simulink model "SecRwLtStCalib"  (R2024b)
settings: Solver=FixedStepDiscrete  StartTime=0.0  StopTime=10.0  FixedStep=0.01  RelTol=1e-3
model workspace (MAT data in the model file):
  KeSMSwAcsMd6SecRwLtStBkReclnUpwdDnwdPos1Max_Val : Simulink.Parameter (value not decoded)
  KeSMSwAcsMd6SecRwLtStBkReclnUpwdDnwdPos1Min_Val : Simulink.Parameter (value not decoded)
  KeSMSwAcsMd6SecRwLtStBkReclnUpwdDnwdPos1_Val : Simulink.Parameter (value not decoded)
  KeSMSwAcsMd6SecRwLtStBkReclnUpwdDnwdPosMax_Val : Simulink.Parameter (value not decoded)
  KeSMSwAcsMd6SecRwLtStBkReclnUpwdDnwdPosMin_Val : Simulink.Parameter (value not decoded)
  KeSMSwAcsMd6SecRwLtStBkReclnUpwdDnwdPos_Val : Simulink.Parameter (value not decoded)
symbols that are objects in the model workspace (value not decoded): KeSMSwAcsMd6SecRwLtStBkReclnUpwdDnwdPos1_Val, KeSMSwAcsMd6SecRwLtStBkReclnUpwdDnwdPos1Max_Val, KeSMSwAcsMd6SecRwLtStBkReclnUpwdDnwdPos1Min_Val, KeSMSwAcsMd6SecRwLtStBkReclnUpwdDnwdPos_Val, KeSMSwAcsMd6SecRwLtStBkReclnUpwdDnwdPosMax_Val, KeSMSwAcsMd6SecRwLtStBkReclnUpwdDnwdPosMin_Val
undefined symbols (not defined in the file or in its folder): KeSMSw4SAcsMd21SecRwLtStBkReclnUpwdDnwdPos_Val, KeSMSw4SAcsMd21SecRwLtStBkReclnUpwdDnwdPosMax_Val, KeSMSw4SAcsMd21SecRwLtStBkReclnUpwdDnwdPosMin_Val, KeSMSw4SAcsMd21SecRwLtStFrwdBkwdPos_Val, KeSMSw4SAcsMd21SecRwLtStFrwdBkwdPosMax_Val, KeSMSw4SAcsMd21SecRwLtStFrwdBkwdPosMin_Val, KeSMSw4SAcsMd21SecRwLtStHdrstFrwdBkwdPos_Val, KeSMSw4SAcsMd21SecRwLtStHdrstFrwdBkwdPosMax_Val, KeSMSw4SAcsMd21SecRwLtStHdrstFrwdBkwdPosMin_Val, KeSMSw4SAcsMd21SecRwLtStHdrstUpwdDnwdPos_Val, KeSMSw4SAcsMd21SecRwLtStHdrstUpwdDnwdPosMax_Val, KeSMSw4SAcsMd21SecRwLtStHdrstUpwdDnwdPosMin_Val, KeSMSw4SAcsMd22SecRwLtStBkReclnUpwdDnwdPos1_Val, KeSMSw4SAcsMd22SecRwLtStBkReclnUpwdDnwdPos2_Val, KeSMSw4SAcsMd22SecRwLtStBkReclnUpwdDnwdPos2Max_Val, KeSMSw4SAcsMd22SecRwLtStBkReclnUpwdDnwdPos2Min_Val, KeSMSw4SAcsMd22SecRwLtStBkReclnUpwdDnwdPosMax_Val, KeSMSw4SAcsMd22SecRwLtStBkReclnUpwdDnwdPosMin_Val, KeSMSw4SAcsMd22SecRwLtStFrwdBkwdPos_Val, KeSMSw4SAcsMd22SecRwLtStFrwdBkwdPosMax_Val, KeSMSw4SAcsMd22SecRwLtStFrwdBkwdPosMin_Val, KeSMSw4SAcsMd22SecRwLtStFtrstUpwdDnwdPos_Val, KeSMSw4SAcsMd22SecRwLtStFtrstUpwdDnwdPosMax_Val, KeSMSw4SAcsMd22SecRwLtStFtrstUpwdDnwdPosMin_Val, KeSMSw4SAcsMd22SecRwLtStHdrstFrwdBkwdPos_Val, KeSMSw4SAcsMd22SecRwLtStHdrstFrwdBkwdPosMax_Val, KeSMSw4SAcsMd22SecRwLtStHdrstFrwdBkwdPosMin_Val, KeSMSw4SAcsMd22SecRwLtStHdrstUpwdDnwdPos_Val, KeSMSw4SAcsMd22SecRwLtStHdrstUpwdDnwdPosMax_Val, KeSMSw4SAcsMd22SecRwLtStHdrstUpwdDnwdPosMin_Val, KeSMSw4SAcsMd22SecRwLtStLegrstOtwdInwdPos_Val, KeSMSw4SAcsMd22SecRwLtStLegrstOtwdInwdPosMax_Val, KeSMSw4SAcsMd22SecRwLtStLegrstOtwdInwdPosMin_Val, KeSMSw4SAcsMd22SecRwLtStLegrstUpwdDnwdPos_Val, KeSMSw4SAcsMd22SecRwLtStLegrstUpwdDnwdPosMax_Val, KeSMSw4SAcsMd22SecRwLtStLegrstUpwdDnwdPosMin_Val, KeSMSw4SAcsMd25SecRwLtStBkReclnUpwdDnwdPos_Val, KeSMSw4SAcsMd25SecRwLtStBkReclnUpwdDnwdPosMax_Val, KeSMSw4SAcsMd25SecRwLtStBkReclnUpwdDnwdPosMin_Val, KeSMSw4SAcsMd25SecRwLtStFrwdBkwdPos_Val, KeSMSw4SAcsMd25SecRwLtStFrwdBkwdPosMax_Val, KeSMSw4SAcsMd25SecRwLtStFrwdBkwdPosMin_Val, KeSMSw4SAcsMd25SecRwLtStHdrstFrwdBkwdPos_Val, KeSMSw4SAcsMd25SecRwLtStHdrstFrwdBkwdPosMax_Val, KeSMSw4SAcsMd25SecRwLtStHdrstFrwdBkwdPosMin_Val, KeSMSw4SAcsMd25SecRwLtStHdrstUpwdDnwdPos_Val, KeSMSw4SAcsMd25SecRwLtStHdrstUpwdDnwdPosMax_Val, KeSMSw4SAcsMd25SecRwLtStHdrstUpwdDnwdPosMin_Val, KeSMSw4SAcsMd26SecRwLtStBkReclnUpwdDnwdPos_Val, KeSMSw4SAcsMd26SecRwLtStBkReclnUpwdDnwdPosMax_Val, KeSMSw4SAcsMd26SecRwLtStBkReclnUpwdDnwdPosMin_Val, KeSMSw4SAcsMd26SecRwLtStFrwdBkwdPos_Val, KeSMSw4SAcsMd26SecRwLtStFrwdBkwdPosMax_Val, KeSMSw4SAcsMd26SecRwLtStFrwdBkwdPosMin_Val, KeSMSw4SAcsMd26SecRwLtStFtrstUpwdDnwdPos_Val, KeSMSw4SAcsMd26SecRwLtStFtrstUpwdDnwdPosMax_Val, KeSMSw4SAcsMd26SecRwLtStFtrstUpwdDnwdPosMin_Val, KeSMSw4SAcsMd26SecRwLtStHdrstFrwdBkwdPos_Val, KeSMSw4SAcsMd26SecRwLtStHdrstFrwdBkwdPosMax_Val, KeSMSw4SAcsMd26SecRwLtStHdrstFrwdBkwdPosMin_Val ... (+496)
libraries: TrgtPosSelcLib x61, StIsPosChkLib x1, simulink x1
(part 5 of 8)

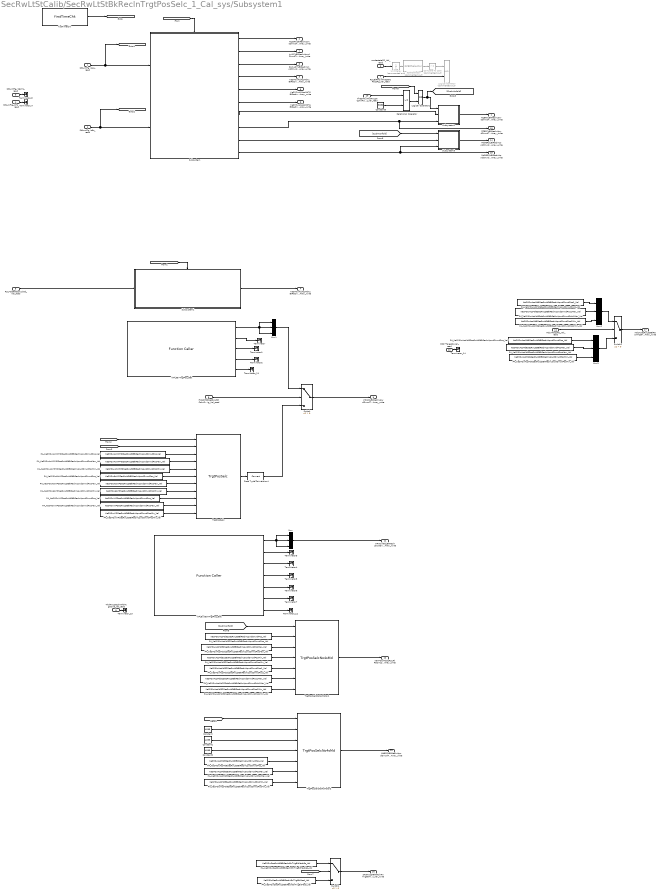
== system SecRwLtStCalib/SecRwLtStBkReclnTrgtPosSelc_1_Cal_sys/Subsystem1 ==
  StNumFlg_Is4s_read : Inport
  StNumFlg_Is6s_read : Inport  Port=2
  StNumFlg_Is6s7s_read : Inport  Port=3
  StNumFlg_Is7s_read : Inport  Port=4
  R2LMdSeatOccupied_Val_read : Inport  Port=5
  modestate32_Val_read : Inport  Port=6
  R2LBkReclinFirstStepPassFlg_Val_read : Inport  Port=7
  IfVeSMSbSecRwLtStCshnFrntUpwdDnwdMovConfig_Val_read : Inport  Port=8
  ThdRwLtStCshnFldStgDone_Val_read : Inport  Port=9
  IfVeSMSuThdRwLtStCshnFldUpwdDnwdPos_Val_read : Inport  Port=10
  Md27Target1_Val_read : Inport  Port=11
  Md27Target2_Val_read : Inport  Port=12
  32BitSelector : StIsPosChkLib/32BitSelector  Commented=on  BitNum=0
  Compare To Zero : simulink/Logic and Bit Operations/Compare To Zero  Commented=on  relop=>  OutDataTypeStr=boolean
  Constant : Constant  Value=4095  OutDataTypeStr=uint16
  Constant1 : Constant  Value=4095  OutDataTypeStr=uint16
  Constant2 : Constant  Value=4095  OutDataTypeStr=uint16
  Constant3 : Constant  Value=3880  OutDataTypeStr=uint16
  Data Type Conversion4 : DataTypeConversion  SaturateOnIntegerOverflow=off  RndMeth=Floor
  Logical Operator : Logic  Commented=on  AllPortsSameDT=off  OutDataTypeStr=boolean
  Logical Operator1 : Logic  Operator=OR  AllPortsSameDT=off  OutDataTypeStr=boolean
  Mux{,1..3} (4 alike) : Mux  Inputs=3
  PA_KeSMSw4sVIPMDSecRwLtStBkReclnUpwdDnwdPosMax_Val : Constant  Value=KeSMSw4sVIPMDSecRwLtStBkReclnUpwdDnwdPosMax_Val
  PA_KeSMSw4sVIPMDSecRwLtStBkReclnUpwdDnwdPosMin_Val : Constant  Value=KeSMSw4sVIPMDSecRwLtStBkReclnUpwdDnwdPosMin_Val
  PA_KeSMSw4sVIPMDSecRwLtStBkReclnUpwdDnwdPos_Val : Constant  Value=KeSMSw4sVIPMDSecRwLtStBkReclnUpwdDnwdPos_Val
  PA_KeSMSw6sVIPSecRwLtStBkReclnUpwdDnwdPosMax_Val : Constant  Value=KeSMSw6sVIPSecRwLtStBkReclnUpwdDnwdPosMax_Val
  PA_KeSMSw6sVIPSecRwLtStBkReclnUpwdDnwdPosMin_Val : Constant  Value=KeSMSw6sVIPSecRwLtStBkReclnUpwdDnwdPosMin_Val
  PA_KeSMSw6sVIPSecRwLtStBkReclnUpwdDnwdPos_Val : Constant  Value=KeSMSw6sVIPSecRwLtStBkReclnUpwdDnwdPos_Val
  PA_KeSMSwAcsMd32SecRwLtStBkReclnUpwdDnwdPos1Max_Val : Constant  Value=KeSMSwAcsMd32SecRwLtStBkReclnUpwdDnwdPos1Max_Val
  PA_KeSMSwAcsMd32SecRwLtStBkReclnUpwdDnwdPos1Min_Val : Constant  Value=KeSMSwAcsMd32SecRwLtStBkReclnUpwdDnwdPos1Min_Val
  PA_KeSMSwAcsMd32SecRwLtStBkReclnUpwdDnwdPos1_Val : Constant  Value=KeSMSwAcsMd32SecRwLtStBkReclnUpwdDnwdPos1_Val
  PA_KeSMSwAcsMd32SecRwLtStBkReclnUpwdDnwdPosMax_Val : Constant  Value=KeSMSwAcsMd32SecRwLtStBkReclnUpwdDnwdPosMax_Val
  PA_KeSMSwAcsMd32SecRwLtStBkReclnUpwdDnwdPosMin_Val : Constant  Value=KeSMSwAcsMd32SecRwLtStBkReclnUpwdDnwdPosMin_Val
  PA_KeSMSwAcsMd32SecRwLtStBkReclnUpwdDnwdPos_Val : Constant  Value=KeSMSwAcsMd32SecRwLtStBkReclnUpwdDnwdPos_Val
  PA_KeSMSwAcsMd6SecRwLtStBkReclnUpwdDnwdPos1Max_Val : Constant  Value=KeSMSwAcsMd6SecRwLtStBkReclnUpwdDnwdPos1Max_Val
  PA_KeSMSwAcsMd6SecRwLtStBkReclnUpwdDnwdPos1Min_Val : Constant  Value=KeSMSwAcsMd6SecRwLtStBkReclnUpwdDnwdPos1Min_Val
  PA_KeSMSwAcsMd6SecRwLtStBkReclnUpwdDnwdPos1_Val : Constant  Value=KeSMSwAcsMd6SecRwLtStBkReclnUpwdDnwdPos1_Val
  PA_KeSMSwAcsMd6SecRwLtStBkReclnUpwdDnwdPosMax_Val : Constant  Value=KeSMSwAcsMd6SecRwLtStBkReclnUpwdDnwdPosMax_Val
  PA_KeSMSwAcsMd6SecRwLtStBkReclnUpwdDnwdPosMin_Val : Constant  Value=KeSMSwAcsMd6SecRwLtStBkReclnUpwdDnwdPosMin_Val
  PA_KeSMSwAcsMd6SecRwLtStBkReclnUpwdDnwdPos_Val : Constant  Value=KeSMSwAcsMd6SecRwLtStBkReclnUpwdDnwdPos_Val
  PA_KeSMSwAcsMd8SecRwLtStBkReclnUpwdDnwdPosMax_Val : Constant  Value=KeSMSwAcsMd8SecRwLtStBkReclnUpwdDnwdPosMax_Val
  PA_KeSMSwAcsMd8SecRwLtStBkReclnUpwdDnwdPosMin_Val : Constant  Value=KeSMSwAcsMd8SecRwLtStBkReclnUpwdDnwdPosMin_Val
  PA_KeSMSwAcsMd8SecRwLtStBkReclnUpwdDnwdPos_Val : Constant  Value=KeSMSwAcsMd8SecRwLtStBkReclnUpwdDnwdPos_Val
  PA_KeSMSwSecRwLtStBkReclnEnTrigBitMask6s_Val : Constant  Value=KeSMSwSecRwLtStBkReclnEnTrigBitMask6s_Val
  PA_KeSMSwSecRwLtStBkReclnEnTrigBitMask_Val : Constant  Value=KeSMSwSecRwLtStBkReclnEnTrigBitMask_Val
  PA_KeSMSwVIPSecRwLtStBkReclnUpwdDnwdPosMax_Val : Constant  Value=KeSMSwVIPSecRwLtStBkReclnUpwdDnwdPosMax_Val
  PA_KeSMSwVIPSecRwLtStBkReclnUpwdDnwdPosMin_Val : Constant  Value=KeSMSwVIPSecRwLtStBkReclnUpwdDnwdPosMin_Val
  PA_KeSMSwVIPSecRwLtStBkReclnUpwdDnwdPos_Val : Constant  Value=KeSMSwVIPSecRwLtStBkReclnUpwdDnwdPos_Val
  Relational Operator : RelationalOperator  OutDataTypeStr=boolean  RndMeth=Simplest  InputSameDT=off
  Subsystem : Subsystem
  Subsystem1 : Subsystem
  Subsystem2 : Subsystem
  Subsystem3 : Subsystem
  Switch : Switch  Criteria=u2 > Threshold  SaturateOnIntegerOverflow=off  InputSameDT=off
  Switch1 : Switch  Criteria=u2 > Threshold  SaturateOnIntegerOverflow=off  InputSameDT=off
  Switch2 : Switch  Criteria=u2 > Threshold  SaturateOnIntegerOverflow=off  InputSameDT=off
  Terminator{,1..7} (8 alike) : Terminator
  Terminator_{3..4,11..14} (6 alike) : Terminator
  TrgtPosSelc : TrgtPosSelcLib/TrgtPosSelc  SystemSampleTime=-1  VariantActivationTime=update diagram  AllowFlexibleInterface=on  Latency=0  AutoFrameSizeCalculation=off
  TrgtPosSelcNot4sMotor1 : TrgtPosSelcLib/TrgtPosSelcNo4sMd  SystemSampleTime=-1  VariantActivationTime=update diagram  AllowFlexibleInterface=on  Latency=0  AutoFrameSizeCalculation=off
  TrgtPosSelcNot4sMotor2 : TrgtPosSelcLib/TrgtPosSelcNo4sMd  SystemSampleTime=-1  VariantActivationTime=update diagram  AllowFlexibleInterface=on  Latency=0  AutoFrameSizeCalculation=off
  Unit Delay : UnitDelay  Commented=on  SampleTime=-1  HasFrameUpgradeWarning=on
  VIPL557TrgtPos_Get : FunctionCaller  FunctionPrototype=[SecRwLtStBkReclnTrgtPos,SecRwLtStZeroTrgtPos,SecRwLtStLgrstUpwdDnwdTrgtPos,SecRwLtStLgrstInwdOtwdTrgtPos,SecRwLtStFwdBkwdTrgtPos] = VIPL557TrgtPos_Get()  InputArgumentSpecifications=<Enter example>  OutputArgumentSpecifications=uint16(1), uint16(1), uint16(1), uint16(1), uint16(1)
  VIPLExit557TrgtPos_Get : FunctionCaller  FunctionPrototype=[SecRwLtStBkReclnTrgtPos,SecRwLtStZeroTrgtPos,SecRwLtStLgrstUpwdDnwdTrgtPos,SecRwLtStLgrstInwdOtwdTrgtPos,ThdRwLtStBkReclnTrgtPos,ThdRwLtStFwdBkwdTrgtPos,SecRwLtStFwdBkwdTrgtPos] = VIPLExit557TrgtPos_Get()  InputArgumentSpecifications=<Enter example>  OutputArgumentSpecifications=uint16(1), uint16(1), uint16(1), uint16(1), uint16(1), uint16(1), uint16(1)
  firstTimeChk : TrgtPosSelcLib/firstTimeChk  SystemSampleTime=-1  VariantActivationTime=update diagram  AllowFlexibleInterface=on  Latency=0  AutoFrameSizeCalculation=off
  EZER2LBkReclnUpwdDnwdTrgtPosCalib_TrgtPosArray_write : Outport  VectorParamsAs1DForOutWhenUnconnected=off
      settings: EnsureOutportIsVirtual=on
  EZQR2LBkReclnUpwdDnwdTrgtPosCalib_TrgtPosArray_write : Outport  Port=2  VectorParamsAs1DForOutWhenUnconnected=off
      settings: EnsureOutportIsVirtual=on
  KeSMSw4SAcsMd21BkReclnUpwdDnwdTrgtPosCalib_TrgtPosArray_write : Outport  Port=3  VectorParamsAs1DForOutWhenUnconnected=off
      settings: EnsureOutportIsVirtual=on
  KeSMSw4SAcsMd22BkReclnUpwdDnwdTrgtPosCalib_TrgtPosArray_write : Outport  Port=4  VectorParamsAs1DForOutWhenUnconnected=off
      settings: EnsureOutportIsVirtual=on
  KeSMSw4SAcsMd25BkReclnUpwdDnwdTrgtPosCalib_TrgtPosArray_write : Outport  Port=5  VectorParamsAs1DForOutWhenUnconnected=off
      settings: EnsureOutportIsVirtual=on
  KeSMSw4SAcsMd26BkReclnUpwdDnwdTrgtPosCalib_TrgtPosArray_write : Outport  Port=6  VectorParamsAs1DForOutWhenUnconnected=off
      settings: EnsureOutportIsVirtual=on
  LyLR2LBkReclnUpwdDnwdTrgtPosCalib_TrgtPosArray_write : Outport  Port=7  VectorParamsAs1DForOutWhenUnconnected=off
      settings: EnsureOutportIsVirtual=on
  RecvLR2LBkReclnUpwdDnwdTrgtPosCalib_TrgtPosArray_write : Outport  Port=8  VectorParamsAs1DForOutWhenUnconnected=off
      settings: EnsureOutportIsVirtual=on
  VIPLR2LBkReclnUpwdDnwdTrgtPosCalib_TrgtPosArray_write : Outport  Port=9  VectorParamsAs1DForOutWhenUnconnected=off
      settings: EnsureOutportIsVirtual=on
  EZER2LBkReclnUpwdDnwdTrgtPosCalib1_TrgtPosArray_write : Outport  Port=10  VectorParamsAs1DForOutWhenUnconnected=off
      settings: EnsureOutportIsVirtual=on
  VIPLExitR2LBkReclnUpwdDnwdTrgtPosCalib_TrgtPosArray_write : Outport  Port=11  VectorParamsAs1DForOutWhenUnconnected=off
      settings: EnsureOutportIsVirtual=on
  KeSMSwMd32R2LBkReclnUpwdDnwdTrgtPosCalib_TrgtPosArray_write : Outport  Port=12  VectorParamsAs1DForOutWhenUnconnected=off
      settings: EnsureOutportIsVirtual=on
  Md8R2LBkReclnUpwdDnwdTrgtPosCalib_TrgtPosArray_write : Outport  Port=13  VectorParamsAs1DForOutWhenUnconnected=off
      settings: EnsureOutportIsVirtual=on
  Md56R2LBkReclnUpwdDnwdTrgtPosCalib_TrgtPosArray_write : Outport  Port=14  VectorParamsAs1DForOutWhenUnconnected=off
      settings: EnsureOutportIsVirtual=on
  Md56R2LBkReclnUpwdDnwdTrgtPosCalib1_TrgtPosArray_write : Outport  Port=15  VectorParamsAs1DForOutWhenUnconnected=off
      settings: EnsureOutportIsVirtual=on
  SecRwLtStBkReclnEnTrigBitMask_Val_write : Outport  Port=16  VectorParamsAs1DForOutWhenUnconnected=off
      settings: EnsureOutportIsVirtual=on
  Md27SecRwLtStBkReclnTrgtPosCalib_TrgtPosArray_write : Outport  Port=17  VectorParamsAs1DForOutWhenUnconnected=off
  wires:
  StNumFlg_Is4s_read/1 -> [is4s], Subsystem/1(StNumFlg_Is4s_read)
  StNumFlg_Is7s_read/1 -> Terminator_4/1
  Subsystem/2(LyLR2LBkReclnUpwdDnwdTrgtPosCalib_TrgtPosArray_write) -> LyLR2LBkReclnUpwdDnwdTrgtPosCalib_TrgtPosArray_write/1
  Subsystem/1(EZQR2LBkReclnUpwdDnwdTrgtPosCalib_TrgtPosArray_write) -> EZQR2LBkReclnUpwdDnwdTrgtPosCalib_TrgtPosArray_write/1
  firstTimeChk/1 -> [firstTimeflg]
  Switch/1 -> VIPLR2LBkReclnUpwdDnwdTrgtPosCalib_TrgtPosArray_write/1
  StNumFlg_Is6s7s_read/1 -> Terminator_3/1
  [firstTimeflg] -> Subsystem/Enable
  StNumFlg_Is6s_read/1 -> [is6s], Subsystem/2(StNumFlg_Is6s_read)
  Subsystem/3(RecvLR2LBkReclnUpwdDnwdTrgtPosCalib_TrgtPosArray_write) -> RecvLR2LBkReclnUpwdDnwdTrgtPosCalib_TrgtPosArray_write/1
  Subsystem/4(KeSMSw4SAcsMd21BkReclnUpwdDnwdTrgtPosCalib_TrgtPosArray_write) -> KeSMSw4SAcsMd21BkReclnUpwdDnwdTrgtPosCalib_TrgtPosArray_write/1
  Subsystem/5(KeSMSw4SAcsMd25BkReclnUpwdDnwdTrgtPosCalib_TrgtPosArray_write) -> KeSMSw4SAcsMd25BkReclnUpwdDnwdTrgtPosCalib_TrgtPosArray_write/1
  Subsystem/6(KeSMSw4SAcsMd26BkReclnUpwdDnwdTrgtPosCalib_TrgtPosArray_write) -> KeSMSw4SAcsMd26BkReclnUpwdDnwdTrgtPosCalib_TrgtPosArray_write/1
  R2LMdSeatOccupied_Val_read/1 -> Subsystem1/1(R2LMdSeatOccupied_Val_read)
  Subsystem1/1(KeSMSw4SAcsMd22BkReclnUpwdDnwdTrgtPosCalib_TrgtPosArray_write) -> KeSMSw4SAcsMd22BkReclnUpwdDnwdTrgtPosCalib_TrgtPosArray_write/1
  [is4s] -> Subsystem1/Enable
  Subsystem/8(EZER2LBkReclnUpwdDnwdTrgtPosCalib1_TrgtPosArray_write) -> EZER2LBkReclnUpwdDnwdTrgtPosCalib1_TrgtPosArray_write/1, Subsystem2/3(Cal1)
  Subsystem/7(EZER2LBkReclnUpwdDnwdTrgtPosCalib_TrgtPosArray_write) -> Subsystem2/2(Cal2)
  Subsystem2/1(EZECal) -> EZER2LBkReclnUpwdDnwdTrgtPosCalib_TrgtPosArray_write/1
  modestate32_Val_read/1 -> Unit Delay/1
  R2LBkReclinFirstStepPassFlg_Val_read/1 -> Logical Operator/2
  Unit Delay/1 -> 32BitSelector/1
  32BitSelector/1 -> Compare To Zero/1
  Compare To Zero/1 -> Logical Operator/1
  PA_KeSMSw6sVIPSecRwLtStBkReclnUpwdDnwdPosMax_Val/1 -> TrgtPosSelc/7
  PA_KeSMSwVIPSecRwLtStBkReclnUpwdDnwdPosMax_Val/1 -> TrgtPosSelc/10
  PA_KeSMSw4sVIPMDSecRwLtStBkReclnUpwdDnwdPos_Val/1 -> TrgtPosSelc/3
  PA_KeSMSw4sVIPMDSecRwLtStBkReclnUpwdDnwdPosMax_Val/1 -> TrgtPosSelc/4
  TrgtPosSelc/1 -> Data Type Conversion4/1
  [is6s] -> TrgtPosSelc/2
  PA_KeSMSw6sVIPSecRwLtStBkReclnUpwdDnwdPos_Val/1 -> TrgtPosSelc/6
  PA_KeSMSw4sVIPMDSecRwLtStBkReclnUpwdDnwdPosMin_Val/1 -> TrgtPosSelc/5
  PA_KeSMSwVIPSecRwLtStBkReclnUpwdDnwdPosMin_Val/1 -> TrgtPosSelc/11
  [is4s] -> TrgtPosSelc/1
  PA_KeSMSw6sVIPSecRwLtStBkReclnUpwdDnwdPosMin_Val/1 -> TrgtPosSelc/8
  PA_KeSMSwVIPSecRwLtStBkReclnUpwdDnwdPos_Val/1 -> TrgtPosSelc/9
  Mux1/1 -> Switch/1
  VIPL557TrgtPos_Get/1 -> Mux1/3, Mux1/2, Mux1/1
  IfVeSMSbSecRwLtStCshnFrntUpwdDnwdMovConfig_Val_read/1 -> Switch/2
  Data Type Conversion4/1 -> Switch/3
  VIPL557TrgtPos_Get/2 -> Terminator/1
  VIPL557TrgtPos_Get/3 -> Terminator1/1
  VIPL557TrgtPos_Get/4 -> Terminator2/1
  Mux/1 -> VIPLExitR2LBkReclnUpwdDnwdTrgtPosCalib_TrgtPosArray_write/1
  VIPLExit557TrgtPos_Get/1 -> Mux/3, Mux/1, Mux/2
  VIPLExit557TrgtPos_Get/2 -> Terminator3/1
  VIPLExit557TrgtPos_Get/4 -> Terminator5/1
  VIPLExit557TrgtPos_Get/3 -> Terminator4/1
  VIPLExit557TrgtPos_Get/5 -> Terminator6/1
  VIPLExit557TrgtPos_Get/6 -> Terminator7/1
  VIPL557TrgtPos_Get/5 -> Terminator_11/1
  VIPLExit557TrgtPos_Get/7 -> Terminator_12/1
  PA_KeSMSwAcsMd32SecRwLtStBkReclnUpwdDnwdPos_Val/1 -> TrgtPosSelcNot4sMotor1/2
  PA_KeSMSwAcsMd32SecRwLtStBkReclnUpwdDnwdPosMax_Val/1 -> TrgtPosSelcNot4sMotor1/3
  PA_KeSMSwAcsMd32SecRwLtStBkReclnUpwdDnwdPosMin_Val/1 -> TrgtPosSelcNot4sMotor1/4
  PA_KeSMSwAcsMd32SecRwLtStBkReclnUpwdDnwdPos1_Val/1 -> TrgtPosSelcNot4sMotor1/5
  PA_KeSMSwAcsMd32SecRwLtStBkReclnUpwdDnwdPos1Max_Val/1 -> TrgtPosSelcNot4sMotor1/6
  PA_KeSMSwAcsMd32SecRwLtStBkReclnUpwdDnwdPos1Min_Val/1 -> TrgtPosSelcNot4sMotor1/7
  TrgtPosSelcNot4sMotor1/1 -> KeSMSwMd32R2LBkReclnUpwdDnwdTrgtPosCalib_TrgtPosArray_write/1
  [is6s] -> TrgtPosSelcNot4sMotor2/1
  PA_KeSMSwAcsMd8SecRwLtStBkReclnUpwdDnwdPosMin_Val/1 -> TrgtPosSelcNot4sMotor2/7
  PA_KeSMSwAcsMd8SecRwLtStBkReclnUpwdDnwdPosMax_Val/1 -> TrgtPosSelcNot4sMotor2/6
  PA_KeSMSwAcsMd8SecRwLtStBkReclnUpwdDnwdPos_Val/1 -> TrgtPosSelcNot4sMotor2/5
  Constant2/1 -> TrgtPosSelcNot4sMotor2/4
  Constant1/1 -> TrgtPosSelcNot4sMotor2/3
  Constant/1 -> TrgtPosSelcNot4sMotor2/2
  TrgtPosSelcNot4sMotor2/1 -> Md8R2LBkReclnUpwdDnwdTrgtPosCalib_TrgtPosArray_write/1
  IfVeSMSuThdRwLtStCshnFldUpwdDnwdPos_Val_read/1 -> Relational Operator/1
  Constant3/1 -> Relational Operator/2
  [CushnUnfold] -> TrgtPosSelcNot4sMotor1/1
  ThdRwLtStCshnFldStgDone_Val_read/1 -> Terminator_13/1
  Subsystem/10(Md56R2LBkReclnUpwdDnwdTrgtPosCalib1_TrgtPosArray_write) -> Subsystem3/3(Cal1), Md56R2LBkReclnUpwdDnwdTrgtPosCalib1_TrgtPosArray_write/1
  Subsystem3/1(EZECal) -> Md56R2LBkReclnUpwdDnwdTrgtPosCalib_TrgtPosArray_write/1
  [CushnUnfold] -> Subsystem3/1(FirstStepPassFlg)
  Subsystem/9(Md56R2LBkReclnUpwdDnwdTrgtPosCalib_TrgtPosArray_write) -> Subsystem3/2(Cal2)
  Switch1/1 -> SecRwLtStBkReclnEnTrigBitMask_Val_write/1
  [is6s] -> Switch1/2
  PA_KeSMSwSecRwLtStBkReclnEnTrigBitMask6s_Val/1 -> Switch1/1
  PA_KeSMSwSecRwLtStBkReclnEnTrigBitMask_Val/1 -> Switch1/3
  Relational Operator/1 -> Logical Operator1/2
  [is6s] -> Logical Operator1/1
  Logical Operator1/1 -> [CushnUnfold], Subsystem2/1(FirstStepPassFlg)
  Md27Target1_Val_read/1 -> Switch2/2
  Mux2/1 -> Switch2/1
  Switch2/1 -> Md27SecRwLtStBkReclnTrgtPosCalib_TrgtPosArray_write/1
  Md27Target2_Val_read/1 -> Terminator_14/1
  PA_KeSMSwAcsMd6SecRwLtStBkReclnUpwdDnwdPos1_Val/1 -> Mux2/1
  PA_KeSMSwAcsMd6SecRwLtStBkReclnUpwdDnwdPos1Max_Val/1 -> Mux2/2
  PA_KeSMSwAcsMd6SecRwLtStBkReclnUpwdDnwdPos1Min_Val/1 -> Mux2/3
  Mux3/1 -> Switch2/3
  PA_KeSMSwAcsMd6SecRwLtStBkReclnUpwdDnwdPos_Val/1 -> Mux3/1
  PA_KeSMSwAcsMd6SecRwLtStBkReclnUpwdDnwdPosMax_Val/1 -> Mux3/2
  PA_KeSMSwAcsMd6SecRwLtStBkReclnUpwdDnwdPosMin_Val/1 -> Mux3/3

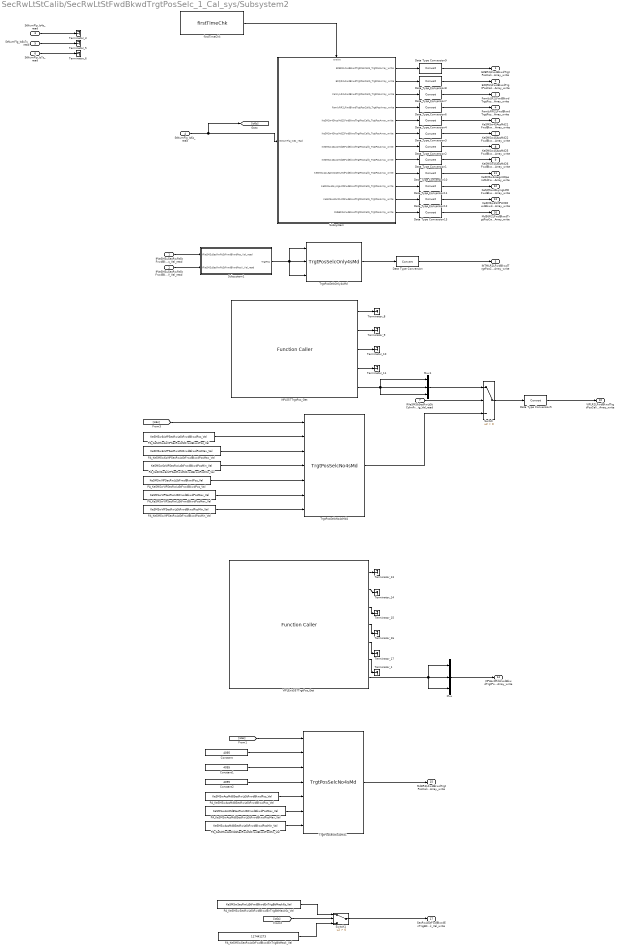
== system SecRwLtStCalib/SecRwLtStFwdBkwdTrgtPosSelc_1_Cal_sys/Subsystem2 ==
  IfVeSMSuSecRwRtStFrwdBkwdPos_Val_read : Inport
  IfVeSMSuSecRwRtStFrwdBkwdPosV_Val_read : Inport  Port=2
  StNumFlg_Is4s_read : Inport  Port=3
  StNumFlg_Is6s_read : Inport  Port=4
  StNumFlg_Is6s7s_read : Inport  Port=5
  StNumFlg_Is7s_read : Inport  Port=6
  IfVeSMSbSecRwLtStCshnFrntUpwdDnwdMovConfig_Val_read : Inport  Port=7
  Constant : Constant  Value=4095  OutDataTypeStr=uint16
  Constant1 : Constant  Value=4095  OutDataTypeStr=uint16
  Constant2 : Constant  Value=4095  OutDataTypeStr=uint16
  Data Type Conversion{,1..13} (14 alike) : DataTypeConversion  SaturateOnIntegerOverflow=off  RndMeth=Floor
  Mux : Mux  Inputs=3
  Mux1 : Mux  Inputs=3
  PA_KeSMSw6sVIPSecRwLtStFrwdBkwdPosMax_Val : Constant  Value=KeSMSw6sVIPSecRwLtStFrwdBkwdPosMax_Val
  PA_KeSMSw6sVIPSecRwLtStFrwdBkwdPosMin_Val : Constant  Value=KeSMSw6sVIPSecRwLtStFrwdBkwdPosMin_Val
  PA_KeSMSw6sVIPSecRwLtStFrwdBkwdPos_Val : Constant  Value=KeSMSw6sVIPSecRwLtStFrwdBkwdPos_Val
  PA_KeSMSwAcsMd8SecRwLtStFrwdBkwdPosMax_Val : Constant  Value=KeSMSwAcsMd8SecRwLtStFrwdBkwdPosMax_Val
  PA_KeSMSwAcsMd8SecRwLtStFrwdBkwdPosMin_Val : Constant  Value=KeSMSwAcsMd8SecRwLtStFrwdBkwdPosMin_Val
  PA_KeSMSwAcsMd8SecRwLtStFrwdBkwdPos_Val : Constant  Value=KeSMSwAcsMd8SecRwLtStFrwdBkwdPos_Val
  PA_KeSMSwSecRwLtStFwdBkwdEnTrigBitMask6s_Val : Constant  Value=KeSMSwSecRwLtStFwdBkwdEnTrigBitMask6s_Val
  PA_KeSMSwSecRwLtStFwdBkwdEnTrigBitMask_Val : Constant  Value=117441273  OutDataTypeStr=uint32
  PA_KeSMSwVIPSecRwLtStFrwdBkwdPosMax_Val : Constant  Value=KeSMSwVIPSecRwLtStFrwdBkwdPosMax_Val
  PA_KeSMSwVIPSecRwLtStFrwdBkwdPosMin_Val : Constant  Value=KeSMSwVIPSecRwLtStFrwdBkwdPosMin_Val
  PA_KeSMSwVIPSecRwLtStFrwdBkwdPos_Val : Constant  Value=KeSMSwVIPSecRwLtStFrwdBkwdPos_Val
  Subsystem : Subsystem
  Subsystem1 : Subsystem
  Switch : Switch  Criteria=u2 > Threshold  SaturateOnIntegerOverflow=off  InputSameDT=off
  Switch1 : Switch  Criteria=u2 > Threshold  SaturateOnIntegerOverflow=off  InputSameDT=off
  Terminator_{1,3,5..6,8..11,13..17} (13 alike) : Terminator
  TrgtPosSelcNo4sMd1 : TrgtPosSelcLib/TrgtPosSelcNo4sMd  SystemSampleTime=-1  VariantActivationTime=update diagram  AllowFlexibleInterface=on  Latency=0  AutoFrameSizeCalculation=off
  TrgtPosSelcNo4sMd4 : TrgtPosSelcLib/TrgtPosSelcNo4sMd  SystemSampleTime=-1  VariantActivationTime=update diagram  AllowFlexibleInterface=on  Latency=0  AutoFrameSizeCalculation=off
  TrgtPosSelcOnly4sMd : TrgtPosSelcLib/TrgtPosSelcOnly4sMd  SystemSampleTime=-1  VariantActivationTime=update diagram  AllowFlexibleInterface=on  Latency=0  AutoFrameSizeCalculation=off
  VIPL557TrgtPos_Get : FunctionCaller  FunctionPrototype=[SecRwLtStBkReclnTrgtPos,SecRwLtStZeroTrgtPos,SecRwLtStLgrstUpwdDnwdTrgtPos,SecRwLtStLgrstInwdOtwdTrgtPos,SecRwLtStFwdBkwdTrgtPos] = VIPL557TrgtPos_Get()  InputArgumentSpecifications=<Enter example>  OutputArgumentSpecifications=uint16(1), uint16(1), uint16(1), uint16(1), uint16(1)
  VIPLExit557TrgtPos_Get : FunctionCaller  FunctionPrototype=[SecRwLtStBkReclnTrgtPos,SecRwLtStZeroTrgtPos,SecRwLtStLgrstUpwdDnwdTrgtPos,SecRwLtStLgrstInwdOtwdTrgtPos,ThdRwLtStBkReclnTrgtPos,ThdRwLtStFwdBkwdTrgtPos,SecRwLtStFwdBkwdTrgtPos] = VIPLExit557TrgtPos_Get()  InputArgumentSpecifications=<Enter example>  OutputArgumentSpecifications=uint16(1), uint16(1), uint16(1), uint16(1), uint16(1), uint16(1), uint16(1)
  firstTimeChk : TrgtPosSelcLib/firstTimeChk  SystemSampleTime=-1  VariantActivationTime=update diagram  AllowFlexibleInterface=on  Latency=0  AutoFrameSizeCalculation=off
  EZER2LFwdBkwdTrgtPosCalib_TrgtPosArray_write : Outport  VectorParamsAs1DForOutWhenUnconnected=off
      settings: EnsureOutportIsVirtual=on
  EZQR2LFwdBkwdTrgtPosCalib_TrgtPosArray_write : Outport  Port=2  VectorParamsAs1DForOutWhenUnconnected=off
      settings: EnsureOutportIsVirtual=on
  FamlyLR2LFwdBkwdTrgtPosCalib_TrgtPosArray_write : Outport  Port=3  VectorParamsAs1DForOutWhenUnconnected=off
      settings: EnsureOutportIsVirtual=on
  FamlyRR2LFwdBkwdTrgtPosCalib_TrgtPosArray_write : Outport  Port=4  VectorParamsAs1DForOutWhenUnconnected=off
      settings: EnsureOutportIsVirtual=on
  INTMLR2LFwdBkwdTrgtPosCalib_TrgtPosArray_write : Outport  Port=5  VectorParamsAs1DForOutWhenUnconnected=off
      settings: EnsureOutportIsVirtual=on
  KeSMSw4SAcsMd21FwdBkwdTrgtPosCalib_TrgtPosArray_write : Outport  Port=6  VectorParamsAs1DForOutWhenUnconnected=off
      settings: EnsureOutportIsVirtual=on
  KeSMSw4SAcsMd22FwdBkwdTrgtPosCalib_TrgtPosArray_write : Outport  Port=7  VectorParamsAs1DForOutWhenUnconnected=off
      settings: EnsureOutportIsVirtual=on
  KeSMSw4SAcsMd25FwdBkwdTrgtPosCalib_TrgtPosArray_write : Outport  Port=8  VectorParamsAs1DForOutWhenUnconnected=off
      settings: EnsureOutportIsVirtual=on
  KeSMSw4SAcsMd26FwdBkwdTrgtPosCalib_TrgtPosArray_write : Outport  Port=9  VectorParamsAs1DForOutWhenUnconnected=off
      settings: EnsureOutportIsVirtual=on
  VIPLR2LFwdBkwdTrgtPosCalib_TrgtPosArray_write : Outport  Port=10  VectorParamsAs1DForOutWhenUnconnected=off
      settings: EnsureOutportIsVirtual=on
  KeSMSw4sLegrstOpenLMdFwdBkwdTrgtPosCalib_TrgtPosArray_write : Outport  Port=11  VectorParamsAs1DForOutWhenUnconnected=off
      settings: EnsureOutportIsVirtual=on
  KeSMSw4SLyingLMDFwdBkwdTrgtPosCalib_TrgtPosArray_write : Outport  Port=12  VectorParamsAs1DForOutWhenUnconnected=off
      settings: EnsureOutportIsVirtual=on
  KeSMSw4SVIPLMDFwdBkwdTrgtPosCalib_TrgtPosArray_write : Outport  Port=13  VectorParamsAs1DForOutWhenUnconnected=off
      settings: EnsureOutportIsVirtual=on
  VIPLExitR2LFwdBkwdTrgtPosCalib_TrgtPosArray_write : Outport  Port=14  VectorParamsAs1DForOutWhenUnconnected=off
      settings: EnsureOutportIsVirtual=on
  Md8R2LFwdBkwdTrgtPosCalib_TrgtPosArray_write : Outport  Port=15  VectorParamsAs1DForOutWhenUnconnected=off
      settings: EnsureOutportIsVirtual=on
  Md56R2LFwdBkwdTrgtPosCalib_TrgtPosArray_write : Outport  Port=16  VectorParamsAs1DForOutWhenUnconnected=off
      settings: EnsureOutportIsVirtual=on
  SecRwLtStFwdBkwdEnTrigBitMask_Val_write : Outport  Port=17  VectorParamsAs1DForOutWhenUnconnected=off
      settings: EnsureOutportIsVirtual=on
  wires:
  Subsystem/1(EZER2LFwdBkwdTrgtPosCalib_TrgtPosArray_write) -> Data Type Conversion9/1
  StNumFlg_Is4s_read/1 -> Terminator_3/1
  Subsystem1/1(TrgtPos) -> TrgtPosSelcOnly4sMd/2, TrgtPosSelcOnly4sMd/1, TrgtPosSelcOnly4sMd/3
  IfVeSMSuSecRwRtStFrwdBkwdPos_Val_read/1 -> Subsystem1/1(IfVeSMSuSecRwRtStFrwdBkwdPos_Val_read)
  Subsystem/3(FamlyLR2LFwdBkwdTrgtPosCalib_TrgtPosArray_write) -> Data Type Conversion7/1
  StNumFlg_Is6s7s_read/1 -> Terminator_5/1
  StNumFlg_Is7s_read/1 -> Terminator_6/1
  Subsystem/4(FamlyRR2LFwdBkwdTrgtPosCalib_TrgtPosArray_write) -> Data Type Conversion6/1
  Switch/1 -> Data Type Conversion5/1
  StNumFlg_Is6s_read/1 -> [is6s], Subsystem/1(StNumFlg_Is6s_read)
  Subsystem/2(EZQR2LFwdBkwdTrgtPosCalib_TrgtPosArray_write) -> Data Type Conversion8/1
  firstTimeChk/1 -> Subsystem/Enable
  TrgtPosSelcOnly4sMd/1 -> Data Type Conversion/1
  IfVeSMSuSecRwRtStFrwdBkwdPosV_Val_read/1 -> Subsystem1/2(IfVeSMSuSecRwRtStFrwdBkwdPosV_Val_read)
  Subsystem/8(KeSMSw4SAcsMd26FwdBkwdTrgtPosCalib_TrgtPosArray_write) -> Data Type Conversion1/1
  Subsystem/7(KeSMSw4SAcsMd25FwdBkwdTrgtPosCalib_TrgtPosArray_write) -> Data Type Conversion2/1
  Subsystem/6(KeSMSw4SAcsMd22FwdBkwdTrgtPosCalib_TrgtPosArray_write) -> Data Type Conversion3/1
  Subsystem/5(KeSMSw4SAcsMd21FwdBkwdTrgtPosCalib_TrgtPosArray_write) -> Data Type Conversion4/1
  Data Type Conversion/1 -> INTMLR2LFwdBkwdTrgtPosCalib_TrgtPosArray_write/1
  Data Type Conversion1/1 -> KeSMSw4SAcsMd26FwdBkwdTrgtPosCalib_TrgtPosArray_write/1
  Data Type Conversion2/1 -> KeSMSw4SAcsMd25FwdBkwdTrgtPosCalib_TrgtPosArray_write/1
  Data Type Conversion3/1 -> KeSMSw4SAcsMd22FwdBkwdTrgtPosCalib_TrgtPosArray_write/1
  Data Type Conversion4/1 -> KeSMSw4SAcsMd21FwdBkwdTrgtPosCalib_TrgtPosArray_write/1
  Data Type Conversion5/1 -> VIPLR2LFwdBkwdTrgtPosCalib_TrgtPosArray_write/1
  Data Type Conversion6/1 -> FamlyRR2LFwdBkwdTrgtPosCalib_TrgtPosArray_write/1
  Data Type Conversion7/1 -> FamlyLR2LFwdBkwdTrgtPosCalib_TrgtPosArray_write/1
  Data Type Conversion8/1 -> EZQR2LFwdBkwdTrgtPosCalib_TrgtPosArray_write/1
  Data Type Conversion9/1 -> EZER2LFwdBkwdTrgtPosCalib_TrgtPosArray_write/1
  Data Type Conversion12/1 -> KeSMSw4SVIPLMDFwdBkwdTrgtPosCalib_TrgtPosArray_write/1
  Data Type Conversion10/1 -> KeSMSw4sLegrstOpenLMdFwdBkwdTrgtPosCalib_TrgtPosArray_write/1
  Data Type Conversion11/1 -> KeSMSw4SLyingLMDFwdBkwdTrgtPosCalib_TrgtPosArray_write/1
  Subsystem/9(KeSMSw4sLegrstOpenLMdFwdBkwdTrgtPosCalib_TrgtPosArray_write) -> Data Type Conversion10/1
  Subsystem/10(KeSMSw4SLyingLMDFwdBkwdTrgtPosCalib_TrgtPosArray_write) -> Data Type Conversion11/1
  Subsystem/11(KeSMSw4SVIPLMDFwdBkwdTrgtPosCalib_TrgtPosArray_write) -> Data Type Conversion12/1
  IfVeSMSbSecRwLtStCshnFrntUpwdDnwdMovConfig_Val_read/1 -> Switch/2
  [is6s] -> TrgtPosSelcNo4sMd4/1
  PA_KeSMSwVIPSecRwLtStFrwdBkwdPos_Val/1 -> TrgtPosSelcNo4sMd4/5
  PA_KeSMSwVIPSecRwLtStFrwdBkwdPosMax_Val/1 -> TrgtPosSelcNo4sMd4/6
  PA_KeSMSw6sVIPSecRwLtStFrwdBkwdPosMin_Val/1 -> TrgtPosSelcNo4sMd4/4
  PA_KeSMSw6sVIPSecRwLtStFrwdBkwdPos_Val/1 -> TrgtPosSelcNo4sMd4/2
  PA_KeSMSwVIPSecRwLtStFrwdBkwdPosMin_Val/1 -> TrgtPosSelcNo4sMd4/7
  PA_KeSMSw6sVIPSecRwLtStFrwdBkwdPosMax_Val/1 -> TrgtPosSelcNo4sMd4/3
  TrgtPosSelcNo4sMd4/1 -> Switch/3
  VIPL557TrgtPos_Get/1 -> Terminator_8/1
  VIPL557TrgtPos_Get/2 -> Terminator_9/1
  VIPL557TrgtPos_Get/3 -> Terminator_10/1
  VIPL557TrgtPos_Get/4 -> Terminator_11/1
  VIPLExit557TrgtPos_Get/1 -> Terminator_13/1
  VIPLExit557TrgtPos_Get/2 -> Terminator_14/1
  VIPLExit557TrgtPos_Get/3 -> Terminator_15/1
  VIPLExit557TrgtPos_Get/4 -> Terminator_16/1
  VIPLExit557TrgtPos_Get/5 -> Terminator_17/1
  Mux/1 -> VIPLExitR2LFwdBkwdTrgtPosCalib_TrgtPosArray_write/1
  Mux1/1 -> Switch/1
  VIPL557TrgtPos_Get/5 -> Mux1/3, Mux1/2, Mux1/1
  VIPLExit557TrgtPos_Get/7 -> Mux/3, Mux/1, Mux/2
  VIPLExit557TrgtPos_Get/6 -> Terminator_1/1
  [is6s] -> TrgtPosSelcNo4sMd1/1
  PA_KeSMSwAcsMd8SecRwLtStFrwdBkwdPos_Val/1 -> TrgtPosSelcNo4sMd1/5
  PA_KeSMSwAcsMd8SecRwLtStFrwdBkwdPosMax_Val/1 -> TrgtPosSelcNo4sMd1/6
  PA_KeSMSwAcsMd8SecRwLtStFrwdBkwdPosMin_Val/1 -> TrgtPosSelcNo4sMd1/7
  TrgtPosSelcNo4sMd1/1 -> Md8R2LFwdBkwdTrgtPosCalib_TrgtPosArray_write/1
  Constant/1 -> TrgtPosSelcNo4sMd1/2
  Constant1/1 -> TrgtPosSelcNo4sMd1/3
  Constant2/1 -> TrgtPosSelcNo4sMd1/4
  Subsystem/12(Md56R2LFwdBkwdTrgtPosCalib_TrgtPosArray_write) -> Data Type Conversion13/1
  Data Type Conversion13/1 -> Md56R2LFwdBkwdTrgtPosCalib_TrgtPosArray_write/1
  Switch1/1 -> SecRwLtStFwdBkwdEnTrigBitMask_Val_write/1
  [is6s] -> Switch1/2
  PA_KeSMSwSecRwLtStFwdBkwdEnTrigBitMask6s_Val/1 -> Switch1/1
  PA_KeSMSwSecRwLtStFwdBkwdEnTrigBitMask_Val/1 -> Switch1/3

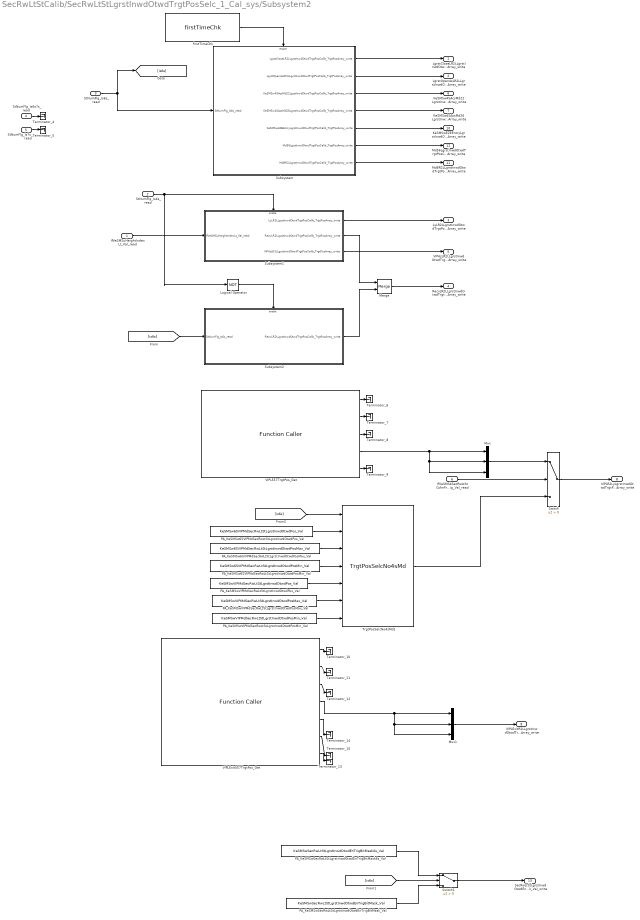
== system SecRwLtStCalib/SecRwLtStLgrstInwdOtwdTrgtPosSelc_1_Cal_sys/Subsystem2 ==
  IfVeSMSuHeightIndexLt_Val_read : Inport
  StNumFlg_Is4s_read : Inport  Port=2
  StNumFlg_Is6s_read : Inport  Port=3
  StNumFlg_Is6s7s_read : Inport  Port=4
  StNumFlg_Is7s_read : Inport  Port=5
  IfVeSMSbSecRwLtStCshnFrntUpwdDnwdMovConfig_Val_read : Inport  Port=6
  Logical Operator : Logic  Operator=NOT  AllPortsSameDT=off  OutDataTypeStr=boolean
  Merge : Merge
  Mux : Mux  Inputs=3
  Mux1 : Mux  Inputs=3
  PA_KeSMSw6SVIPMdSecRwLtStLgrstInwdOtwdPosMax_Val : Constant  Value=KeSMSw6SVIPMdSecRwLtStLgrstInwdOtwdPosMax_Val
  PA_KeSMSw6SVIPMdSecRwLtStLgrstInwdOtwdPosMin_Val : Constant  Value=KeSMSw6SVIPMdSecRwLtStLgrstInwdOtwdPosMin_Val
  PA_KeSMSw6SVIPMdSecRwLtStLgrstInwdOtwdPos_Val : Constant  Value=KeSMSw6SVIPMdSecRwLtStLgrstInwdOtwdPos_Val
  PA_KeSMSwSecRwLtStLgrstInwdOtwdEnTrigBitMask6s_Val : Constant  Value=KeSMSwSecRwLtStLgrstInwdOtwdEnTrigBitMask6s_Val
  PA_KeSMSwSecRwLtStLgrstInwdOtwdEnTrigBitMask_Val : Constant  Value=KeSMSwSecRwLtStLgrstInwdOtwdEnTrigBitMask_Val
  PA_KeSMSwVIPMdSecRwLtStLgrstInwdOtwdPosMax_Val : Constant  Value=KeSMSwVIPMdSecRwLtStLgrstInwdOtwdPosMax_Val
  PA_KeSMSwVIPMdSecRwLtStLgrstInwdOtwdPosMin_Val : Constant  Value=KeSMSwVIPMdSecRwLtStLgrstInwdOtwdPosMin_Val
  PA_KeSMSwVIPMdSecRwLtStLgrstInwdOtwdPos_Val : Constant  Value=KeSMSwVIPMdSecRwLtStLgrstInwdOtwdPos_Val
  Subsystem : Subsystem
  Subsystem1 : Subsystem
  Subsystem2 : Subsystem
  Switch : Switch  Criteria=u2 > Threshold  SaturateOnIntegerOverflow=off  InputSameDT=off
  Switch1 : Switch  Criteria=u2 > Threshold  SaturateOnIntegerOverflow=off  InputSameDT=off
  Terminator_{4..15} (12 alike) : Terminator
  TrgtPosSelcNo4sMd1 : TrgtPosSelcLib/TrgtPosSelcNo4sMd  SystemSampleTime=-1  VariantActivationTime=update diagram  AllowFlexibleInterface=on  Latency=0  AutoFrameSizeCalculation=off
  VIPL557TrgtPos_Get : FunctionCaller  FunctionPrototype=[SecRwLtStBkReclnTrgtPos,SecRwLtStZeroTrgtPos,SecRwLtStLgrstUpwdDnwdTrgtPos,SecRwLtStLgrstInwdOtwdTrgtPos,SecRwLtStFwdBkwdTrgtPos] = VIPL557TrgtPos_Get()  InputArgumentSpecifications=<Enter example>  OutputArgumentSpecifications=uint16(1), uint16(1), uint16(1), uint16(1), uint16(1)
  VIPLExit557TrgtPos_Get : FunctionCaller  FunctionPrototype=[SecRwLtStBkReclnTrgtPos,SecRwLtStZeroTrgtPos,SecRwLtStLgrstUpwdDnwdTrgtPos,SecRwLtStLgrstInwdOtwdTrgtPos,ThdRwLtStBkReclnTrgtPos,ThdRwLtStFwdBkwdTrgtPos,SecRwLtStFwdBkwdTrgtPos] = VIPLExit557TrgtPos_Get()  InputArgumentSpecifications=<Enter example>  OutputArgumentSpecifications=uint16(1), uint16(1), uint16(1), uint16(1), uint16(1), uint16(1), uint16(1)
  firstTimeChk : TrgtPosSelcLib/firstTimeChk  SystemSampleTime=-1  VariantActivationTime=update diagram  AllowFlexibleInterface=on  Latency=0  AutoFrameSizeCalculation=off
  LgrstCloseLR2LLgrstInwdOtwdTrgtPosCalib_TrgtPosArray_write : Outport  VectorParamsAs1DForOutWhenUnconnected=off
      settings: EnsureOutportIsVirtual=on
  LgrstOpen4sLR2LLgrstInwdOtwdTrgtPosCalib_TrgtPosArray_write : Outport  Port=2  VectorParamsAs1DForOutWhenUnconnected=off
      settings: EnsureOutportIsVirtual=on
  LyLR2LLgrstInwdOtwdTrgtPosCalib_TrgtPosArray_write : Outport  Port=3  VectorParamsAs1DForOutWhenUnconnected=off
      settings: EnsureOutportIsVirtual=on
  RecvLR2LLgrstInwdOtwdTrgtPosCalib_TrgtPosArray_write : Outport  Port=4  VectorParamsAs1DForOutWhenUnconnected=off
      settings: EnsureOutportIsVirtual=on
  VIP4sLR2LLgrstInwdOtwdTrgtPosCalib_TrgtPosArray_write : Outport  Port=5  VectorParamsAs1DForOutWhenUnconnected=off
      settings: EnsureOutportIsVirtual=on
  KeSMSw4SAcsMd22LgrstInwdOtwdTrgtPosCalib_TrgtPosArray_write : Outport  Port=6  VectorParamsAs1DForOutWhenUnconnected=off
      settings: EnsureOutportIsVirtual=on
  KeSMSw4SAcsMd26LgrstInwdOtwdTrgtPosCalib_TrgtPosArray_write : Outport  Port=7  VectorParamsAs1DForOutWhenUnconnected=off
      settings: EnsureOutportIsVirtual=on
  VIPLR2LyLgrstInwdOtwdTrgtPosCalib_TrgtPosArray_write : Outport  Port=8  VectorParamsAs1DForOutWhenUnconnected=off
      settings: EnsureOutportIsVirtual=on
  VIPLExitR2LLgrstInwdOtwdTrgtPosCalib_TrgtPosArray_write : Outport  Port=9  VectorParamsAs1DForOutWhenUnconnected=off
      settings: EnsureOutportIsVirtual=on
  KeSMSwEZEEntryLgrstInwdOtwdTrgtPosCalib_TrgtPosArray_write : Outport  Port=10  VectorParamsAs1DForOutWhenUnconnected=off
      settings: EnsureOutportIsVirtual=on
  Md8R2LLgrstInwdOtwdTrgtPosCalib_TrgtPosArray_write : Outport  Port=11  VectorParamsAs1DForOutWhenUnconnected=off
      settings: EnsureOutportIsVirtual=on
  Md56LgrstInwdOtwdTrgtPosCalib_TrgtPosArray_write : Outport  Port=12  VectorParamsAs1DForOutWhenUnconnected=off
      settings: EnsureOutportIsVirtual=on
  SecRwLtStLgrstInwdOtwdEnTrigBitMask_Val_write : Outport  Port=13  VectorParamsAs1DForOutWhenUnconnected=off
      settings: EnsureOutportIsVirtual=on
  wires:
  StNumFlg_Is7s_read/1 -> Terminator_5/1
  Subsystem/2(LgrstOpen4sLR2LLgrstInwdOtwdTrgtPosCalib_TrgtPosArray_write) -> LgrstOpen4sLR2LLgrstInwdOtwdTrgtPosCalib_TrgtPosArray_write/1
  Subsystem1/1(LyLR2LLgrstInwdOtwdTrgtPosCalib_TrgtPosArray_write) -> LyLR2LLgrstInwdOtwdTrgtPosCalib_TrgtPosArray_write/1
  Subsystem/1(LgrstCloseLR2LLgrstInwdOtwdTrgtPosCalib_TrgtPosArray_write) -> LgrstCloseLR2LLgrstInwdOtwdTrgtPosCalib_TrgtPosArray_write/1
  StNumFlg_Is4s_read/1 -> Logical Operator/1, Subsystem1/Enable
  firstTimeChk/1 -> Subsystem/Enable
  StNumFlg_Is6s7s_read/1 -> Terminator_4/1
  Subsystem1/3(VIP4sLR2LLgrstInwdOtwdTrgtPosCalib_TrgtPosArray_write) -> VIP4sLR2LLgrstInwdOtwdTrgtPosCalib_TrgtPosArray_write/1
  IfVeSMSuHeightIndexLt_Val_read/1 -> Subsystem1/1(IfVeSMSuHeightIndexLt_Val_read)
  StNumFlg_Is6s_read/1 -> [is6s], Subsystem/1(StNumFlg_Is6s_read)
  Subsystem/4(KeSMSw4SAcsMd26LgrstInwdOtwdTrgtPosCalib_TrgtPosArray_write) -> KeSMSw4SAcsMd26LgrstInwdOtwdTrgtPosCalib_TrgtPosArray_write/1
  Subsystem/3(KeSMSw4SAcsMd22LgrstInwdOtwdTrgtPosCalib_TrgtPosArray_write) -> KeSMSw4SAcsMd22LgrstInwdOtwdTrgtPosCalib_TrgtPosArray_write/1
  Logical Operator/1 -> Subsystem2/Enable
  [is6s] -> Subsystem2/1(StNumFlg_Is6s_read)
  Subsystem2/1(RecvLR2LLgrstInwdOtwdTrgtPosCalib_TrgtPosArray_write) -> Merge/2
  Subsystem1/2(RecvLR2LLgrstInwdOtwdTrgtPosCalib_TrgtPosArray_write) -> Merge/1
  Merge/1 -> RecvLR2LLgrstInwdOtwdTrgtPosCalib_TrgtPosArray_write/1
  Switch/1 -> VIPLR2LyLgrstInwdOtwdTrgtPosCalib_TrgtPosArray_write/1
  IfVeSMSbSecRwLtStCshnFrntUpwdDnwdMovConfig_Val_read/1 -> Switch/2
  Mux/1 -> Switch/1
  VIPL557TrgtPos_Get/4 -> Mux/1, Mux/3, Mux/2
  VIPL557TrgtPos_Get/1 -> Terminator_6/1
  VIPL557TrgtPos_Get/2 -> Terminator_7/1
  VIPL557TrgtPos_Get/3 -> Terminator_8/1
  VIPL557TrgtPos_Get/5 -> Terminator_9/1
  VIPLExit557TrgtPos_Get/1 -> Terminator_10/1
  VIPLExit557TrgtPos_Get/2 -> Terminator_11/1
  VIPLExit557TrgtPos_Get/3 -> Terminator_12/1
  VIPLExit557TrgtPos_Get/5 -> Terminator_14/1
  VIPLExit557TrgtPos_Get/6 -> Terminator_15/1
  Mux1/1 -> VIPLExitR2LLgrstInwdOtwdTrgtPosCalib_TrgtPosArray_write/1
  VIPLExit557TrgtPos_Get/4 -> Mux1/2, Mux1/3, Mux1/1
  Subsystem/5(KeSMSwEZEEntryLgrstInwdOtwdTrgtPosCalib_TrgtPosArray_write) -> KeSMSwEZEEntryLgrstInwdOtwdTrgtPosCalib_TrgtPosArray_write/1
  VIPLExit557TrgtPos_Get/7 -> Terminator_13/1
  TrgtPosSelcNo4sMd1/1 -> Switch/3
  [is6s] -> TrgtPosSelcNo4sMd1/1
  PA_KeSMSw6SVIPMdSecRwLtStLgrstInwdOtwdPosMax_Val/1 -> TrgtPosSelcNo4sMd1/3
  PA_KeSMSw6SVIPMdSecRwLtStLgrstInwdOtwdPosMin_Val/1 -> TrgtPosSelcNo4sMd1/4
  PA_KeSMSw6SVIPMdSecRwLtStLgrstInwdOtwdPos_Val/1 -> TrgtPosSelcNo4sMd1/2
  PA_KeSMSwVIPMdSecRwLtStLgrstInwdOtwdPosMax_Val/1 -> TrgtPosSelcNo4sMd1/6
  PA_KeSMSwVIPMdSecRwLtStLgrstInwdOtwdPos_Val/1 -> TrgtPosSelcNo4sMd1/5
  PA_KeSMSwVIPMdSecRwLtStLgrstInwdOtwdPosMin_Val/1 -> TrgtPosSelcNo4sMd1/7
  Subsystem/6(Md56LgrstInwdOtwdTrgtPosCalib_TrgtPosArray_write) -> Md56LgrstInwdOtwdTrgtPosCalib_TrgtPosArray_write/1
  Subsystem/7(Md8R2LLgrstInwdOtwdTrgtPosCalib_TrgtPosArray_write) -> Md8R2LLgrstInwdOtwdTrgtPosCalib_TrgtPosArray_write/1
  Switch1/1 -> SecRwLtStLgrstInwdOtwdEnTrigBitMask_Val_write/1
  [is6s] -> Switch1/2
  PA_KeSMSwSecRwLtStLgrstInwdOtwdEnTrigBitMask6s_Val/1 -> Switch1/1
  PA_KeSMSwSecRwLtStLgrstInwdOtwdEnTrigBitMask_Val/1 -> Switch1/3

== system SecRwLtStCalib/SecRwLtStLgrstUpwdDnwdTrgtPosSelc_1_Cal_sys/Subsystem1 ==
  StNumFlg_Is4s_read : Inport
  StNumFlg_Is6s_read : Inport  Port=2
  StNumFlg_Is6s7s_read : Inport  Port=3
  StNumFlg_Is7s_read : Inport  Port=4
  IfVeSMSbSecRwLtStCshnFrntUpwdDnwdMovConfig_Val_read : Inport  Port=5
  Data Type Conversion2 : DataTypeConversion  SaturateOnIntegerOverflow=off  RndMeth=Floor
  Mux : Mux  Inputs=3
  Mux1 : Mux  Inputs=3
  PA_KeSMSw4sVIPMDSecRwLtStLgrstUpwdDnwdPosMax_Val : Constant  Value=KeSMSw4sVIPMDSecRwLtStLgrstUpwdDnwdPosMax_Val
  PA_KeSMSw4sVIPMDSecRwLtStLgrstUpwdDnwdPosMin_Val : Constant  Value=KeSMSw4sVIPMDSecRwLtStLgrstUpwdDnwdPosMin_Val
  PA_KeSMSw4sVIPMDSecRwLtStLgrstUpwdDnwdPos_Val : Constant  Value=KeSMSw4sVIPMDSecRwLtStLgrstUpwdDnwdPos_Val
  PA_KeSMSw6sVIPSecRwLtStLgrstUpwdPosMax_Val : Constant  Value=KeSMSw6sVIPSecRwLtStLgrstUpwdPosMax_Val
  PA_KeSMSw6sVIPSecRwLtStLgrstUpwdPosMin_Val : Constant  Value=KeSMSw6sVIPSecRwLtStLgrstUpwdPosMin_Val
  PA_KeSMSw6sVIPSecRwLtStLgrstUpwdPos_Val : Constant  Value=KeSMSw6sVIPSecRwLtStLgrstUpwdPos_Val
  PA_KeSMSwSecRwLtStLgrstUpwdDnwdEnTrigBitMask6s_Val : Constant  Value=KeSMSwSecRwLtStLgrstUpwdDnwdEnTrigBitMask6s_Val
  PA_KeSMSwSecRwLtStLgrstUpwdDnwdEnTrigBitMask_Val : Constant  Value=KeSMSwSecRwLtStLgrstUpwdDnwdEnTrigBitMask_Val
  PA_KeSMSwVIPSecRwLtStLgrstUpwdPosMax_Val : Constant  Value=KeSMSwVIPSecRwLtStLgrstUpwdPosMax_Val
  PA_KeSMSwVIPSecRwLtStLgrstUpwdPosMin_Val : Constant  Value=KeSMSwVIPSecRwLtStLgrstUpwdPosMin_Val
  PA_KeSMSwVIPSecRwLtStLgrstUpwdPos_Val : Constant  Value=KeSMSwVIPSecRwLtStLgrstUpwdPos_Val
  Subsystem : Subsystem
  Switch : Switch  Criteria=u2 > Threshold  SaturateOnIntegerOverflow=off  InputSameDT=off
  Switch1 : Switch  Criteria=u2 > Threshold  SaturateOnIntegerOverflow=off  InputSameDT=off
  Terminator_{1,3..13} (12 alike) : Terminator
  TrgtPosSelc1 : TrgtPosSelcLib/TrgtPosSelc  SystemSampleTime=-1  VariantActivationTime=update diagram  AllowFlexibleInterface=on  Latency=0  AutoFrameSizeCalculation=off
  VIPL557TrgtPos_Get : FunctionCaller  FunctionPrototype=[SecRwLtStBkReclnTrgtPos,SecRwLtStZeroTrgtPos,SecRwLtStLgrstUpwdDnwdTrgtPos,SecRwLtStLgrstInwdOtwdTrgtPos,SecRwLtStFwdBkwdTrgtPos] = VIPL557TrgtPos_Get()  InputArgumentSpecifications=<Enter example>  OutputArgumentSpecifications=uint16(1), uint16(1), uint16(1), uint16(1), uint16(1)
  VIPLExit557TrgtPos_Get : FunctionCaller  FunctionPrototype=[SecRwLtStBkReclnTrgtPos,SecRwLtStZeroTrgtPos,SecRwLtStLgrstUpwdDnwdTrgtPos,SecRwLtStLgrstInwdOtwdTrgtPos,ThdRwLtStBkReclnTrgtPos,ThdRwLtStFwdBkwdTrgtPos,SecRwLtStFwdBkwdTrgtPos] = VIPLExit557TrgtPos_Get()  InputArgumentSpecifications=<Enter example>  OutputArgumentSpecifications=uint16(1), uint16(1), uint16(1), uint16(1), uint16(1), uint16(1), uint16(1)
  firstTimeChk : TrgtPosSelcLib/firstTimeChk  SystemSampleTime=-1  VariantActivationTime=update diagram  AllowFlexibleInterface=on  Latency=0  AutoFrameSizeCalculation=off
  EZER2LLgrstUpwdDnwdTrgtPosCalib_TrgtPosArray_write : Outport  VectorParamsAs1DForOutWhenUnconnected=off
      settings: EnsureOutportIsVirtual=on
  EZQR2LLgrstUpwdDnwdTrgtPosCalib_TrgtPosArray_write : Outport  Port=2  VectorParamsAs1DForOutWhenUnconnected=off
      settings: EnsureOutportIsVirtual=on
  LgrstCloseLR2LLgrstUpwdDnwdTrgtPosCalib_TrgtPosArray_write : Outport  Port=3  VectorParamsAs1DForOutWhenUnconnected=off
      settings: EnsureOutportIsVirtual=on
  LgrstOpenLR2LLgrstUpwdDnwdTrgtPosCalib_TrgtPosArray_write : Outport  Port=4  VectorParamsAs1DForOutWhenUnconnected=off
      settings: EnsureOutportIsVirtual=on
  LyLR2LLgrstUpwdDnwdTrgtPosCalib_TrgtPosArray_write : Outport  Port=5  VectorParamsAs1DForOutWhenUnconnected=off
      settings: EnsureOutportIsVirtual=on
  RecvLR2LLgrstUpwdDnwdTrgtPosCalib_TrgtPosArray_write : Outport  Port=6  VectorParamsAs1DForOutWhenUnconnected=off
      settings: EnsureOutportIsVirtual=on
  VIPLR2LLgrstUpwdDnwdTrgtPosCalib_TrgtPosArray_write : Outport  Port=7  VectorParamsAs1DForOutWhenUnconnected=off
      settings: EnsureOutportIsVirtual=on
  KeSMSw4SAcsMd22LgrstUpwdDnwdTrgtPosCalib_TrgtPosArray_write : Outport  Port=8  VectorParamsAs1DForOutWhenUnconnected=off
      settings: EnsureOutportIsVirtual=on
  KeSMSw4SAcsMd26LgrstUpwdDnwdTrgtPosCalib_TrgtPosArray_write : Outport  Port=9  VectorParamsAs1DForOutWhenUnconnected=off
      settings: EnsureOutportIsVirtual=on
  VIPExitLR2LLgrstUpwdDnwdTrgtPosCalib_TrgtPosArray_write : Outport  Port=10  VectorParamsAs1DForOutWhenUnconnected=off
      settings: EnsureOutportIsVirtual=on
  Md8R2LLgrstUpwdDnwdTrgtPosCalib_TrgtPosArray_write : Outport  Port=11  VectorParamsAs1DForOutWhenUnconnected=off
      settings: EnsureOutportIsVirtual=on
  Md56R2LLgrstUpwdDnwdTrgtPosCalib_TrgtPosArray_write : Outport  Port=12  VectorParamsAs1DForOutWhenUnconnected=off
      settings: EnsureOutportIsVirtual=on
  SecRwLtStLgrstUpwdDnwdEnTrigBitMask_Val_write : Outport  Port=13  VectorParamsAs1DForOutWhenUnconnected=off
      settings: EnsureOutportIsVirtual=on
  wires:
  Subsystem/6(RecvLR2LLgrstUpwdDnwdTrgtPosCalib_TrgtPosArray_write) -> RecvLR2LLgrstUpwdDnwdTrgtPosCalib_TrgtPosArray_write/1
  Subsystem/4(LgrstOpenLR2LLgrstUpwdDnwdTrgtPosCalib_TrgtPosArray_write) -> LgrstOpenLR2LLgrstUpwdDnwdTrgtPosCalib_TrgtPosArray_write/1
  StNumFlg_Is6s_read/1 -> [Is6s], Subsystem/2(StNumFlg_Is6s_read)
  firstTimeChk/1 -> Subsystem/Enable
  Subsystem/3(LgrstCloseLR2LLgrstUpwdDnwdTrgtPosCalib_TrgtPosArray_write) -> LgrstCloseLR2LLgrstUpwdDnwdTrgtPosCalib_TrgtPosArray_write/1
  Subsystem/2(EZQR2LLgrstUpwdDnwdTrgtPosCalib_TrgtPosArray_write) -> EZQR2LLgrstUpwdDnwdTrgtPosCalib_TrgtPosArray_write/1
  StNumFlg_Is6s7s_read/1 -> Terminator_3/1
  Subsystem/5(LyLR2LLgrstUpwdDnwdTrgtPosCalib_TrgtPosArray_write) -> LyLR2LLgrstUpwdDnwdTrgtPosCalib_TrgtPosArray_write/1
  Subsystem/1(EZER2LLgrstUpwdDnwdTrgtPosCalib_TrgtPosArray_write) -> EZER2LLgrstUpwdDnwdTrgtPosCalib_TrgtPosArray_write/1
  StNumFlg_Is7s_read/1 -> Terminator_4/1
  StNumFlg_Is4s_read/1 -> [Is4s], Subsystem/1(StNumFlg_Is4s_read)
  Subsystem/7(KeSMSw4SAcsMd22LgrstUpwdDnwdTrgtPosCalib_TrgtPosArray_write) -> KeSMSw4SAcsMd22LgrstUpwdDnwdTrgtPosCalib_TrgtPosArray_write/1
  Subsystem/8(KeSMSw4SAcsMd26LgrstUpwdDnwdTrgtPosCalib_TrgtPosArray_write) -> KeSMSw4SAcsMd26LgrstUpwdDnwdTrgtPosCalib_TrgtPosArray_write/1
  PA_KeSMSwVIPSecRwLtStLgrstUpwdPos_Val/1 -> TrgtPosSelc1/9
  PA_KeSMSw4sVIPMDSecRwLtStLgrstUpwdDnwdPosMin_Val/1 -> TrgtPosSelc1/5
  PA_KeSMSwVIPSecRwLtStLgrstUpwdPosMin_Val/1 -> TrgtPosSelc1/11
  PA_KeSMSw6sVIPSecRwLtStLgrstUpwdPosMin_Val/1 -> TrgtPosSelc1/8
  PA_KeSMSw6sVIPSecRwLtStLgrstUpwdPosMax_Val/1 -> TrgtPosSelc1/7
  PA_KeSMSw4sVIPMDSecRwLtStLgrstUpwdDnwdPosMax_Val/1 -> TrgtPosSelc1/4
  PA_KeSMSw4sVIPMDSecRwLtStLgrstUpwdDnwdPos_Val/1 -> TrgtPosSelc1/3
  TrgtPosSelc1/1 -> Data Type Conversion2/1
  [Is4s] -> TrgtPosSelc1/1
  PA_KeSMSwVIPSecRwLtStLgrstUpwdPosMax_Val/1 -> TrgtPosSelc1/10
  PA_KeSMSw6sVIPSecRwLtStLgrstUpwdPos_Val/1 -> TrgtPosSelc1/6
  [Is6s] -> TrgtPosSelc1/2
  IfVeSMSbSecRwLtStCshnFrntUpwdDnwdMovConfig_Val_read/1 -> Switch/2
  Data Type Conversion2/1 -> Switch/3
  Switch/1 -> VIPLR2LLgrstUpwdDnwdTrgtPosCalib_TrgtPosArray_write/1
  Mux/1 -> Switch/1
  VIPL557TrgtPos_Get/3 -> Mux/3, Mux/1, Mux/2
  Mux1/1 -> VIPExitLR2LLgrstUpwdDnwdTrgtPosCalib_TrgtPosArray_write/1
  VIPL557TrgtPos_Get/1 -> Terminator_5/1
  VIPL557TrgtPos_Get/2 -> Terminator_6/1
  VIPL557TrgtPos_Get/4 -> Terminator_7/1
  VIPL557TrgtPos_Get/5 -> Terminator_8/1
  VIPLExit557TrgtPos_Get/1 -> Terminator_9/1
  VIPLExit557TrgtPos_Get/2 -> Terminator_10/1
  VIPLExit557TrgtPos_Get/4 -> Terminator_11/1
  VIPLExit557TrgtPos_Get/5 -> Terminator_12/1
  VIPLExit557TrgtPos_Get/6 -> Terminator_13/1
  VIPLExit557TrgtPos_Get/7 -> Terminator_1/1
  VIPLExit557TrgtPos_Get/3 -> Mux1/1, Mux1/3, Mux1/2
  Subsystem/9(Md56R2LLgrstUpwdDnwdTrgtPosCalib_TrgtPosArray_write) -> Md56R2LLgrstUpwdDnwdTrgtPosCalib_TrgtPosArray_write/1
  Subsystem/10(Md8R2LLgrstUpwdDnwdTrgtPosCalib_TrgtPosArray_write) -> Md8R2LLgrstUpwdDnwdTrgtPosCalib_TrgtPosArray_write/1
  [Is6s] -> Switch1/2
  PA_KeSMSwSecRwLtStLgrstUpwdDnwdEnTrigBitMask6s_Val/1 -> Switch1/1
  PA_KeSMSwSecRwLtStLgrstUpwdDnwdEnTrigBitMask_Val/1 -> Switch1/3
  Switch1/1 -> SecRwLtStLgrstUpwdDnwdEnTrigBitMask_Val_write/1
